simulink library "Simple_lib"  (R2018b)
settings: Solver=ode45  StartTime=0.0  StopTime=10.0  RelTol=1e-3  EnableMultiTasking=on
undefined symbols (not defined in the file or in its folder): Acceptance, beta, C, C_J, C_P, c_wall, dGain, DiscIntNeverNeededParam, Duplex, Electrical_lib, grab, h_fe, i, i3, K_T, Kman, KmanCE, mu_s, n_rev, R_arm, Simplex, systemTs, tau_0, TinIC, Ts, w_0, wallMass, Watch_lib
libraries: $bdroot x407, PlantUtilityBlockset_lib x30, peGeneralControl x22, simulink x11
(part 12 of 14)

== system Simple_lib/Hydraulic/Quadratic Heat Pipe/Push ==
  InPot : Inport
  InFlow : Inport  Tag=NOFLUX  Port=2
  FlowDisplay : Display
  Flow_PushO1BoxIIValveHydroNonStandard : Scope
      settings: Tag=Flow
  PotDisplay : Display
  Pot_PushO1BoxIIValveHydroNonStandard : Scope
      settings: Tag=Pot
  Rate Transition : RateTransition  OutPortSampleTimeMultiple=Ts  OutPortSampleTime=Ts
  OutPot : Outport  Tag=NOFLUX
  tag scope: PushO1BoxIIValveHydroNonStandard=global
  wires:
  Rate Transition/1 -> PotDisplay/1, Pot_PushO1BoxIIValveHydroNonStandard/1, OutPot/1
  InFlow/1 -> [PushO1BoxIIValveHydroNonStandard], FlowDisplay/1, Flow_PushO1BoxIIValveHydroNonStandard/1
  InPot/1 -> Rate Transition/1

== system Simple_lib/Hydraulic/Quadratic Pipe/Pull ==
  InPot : Inport  Tag=NOFLUX
  FlowDisplay : Display
  FlowGain : Gain
  FlowSum : Sum  Inputs=2  SaturateOnIntegerOverflow=on  InputSameDT=on  OutDataTypeStr=Inherit: Same as first input
  Flow_PullO1BoxIIValveHydroNonStandard : Scope
      settings: Tag=Flow
  PotDisplay : Display
  Pot_PullO1BoxIIValveHydroNonStandard : Scope
      settings: Tag=Pot
  Rate Transition : RateTransition  OutPortSampleTimeMultiple=nT  OutPortSampleTime=Ts
  OutPot : Outport
  OutFlow : Outport  Tag=NOFLUX  Port=2
  wires:
  Rate Transition/1 -> OutPot/1
  InPot/1 -> Rate Transition/1, PotDisplay/1, Pot_PullO1BoxIIValveHydroNonStandard/1
  FlowGain/1 -> OutFlow/1, Flow_PullO1BoxIIValveHydroNonStandard/1, FlowDisplay/1
  FlowSum/1 -> FlowGain/1
  [PushO3BoxXValveHydroNonStandard] -> FlowSum/1
  [PushInertiaChamber1CylinderHydroNonStandard] -> FlowSum/2

== system Simple_lib/Hydraulic/Quadratic Pipe/Push ==
  InPot : Inport
  InFlow : Inport  Tag=NOFLUX  Port=2
  FlowDisplay : Display
  Flow_PushO1BoxIIValveHydroNonStandard : Scope
      settings: Tag=Flow
  PotDisplay : Display
  Pot_PushO1BoxIIValveHydroNonStandard : Scope
      settings: Tag=Pot
  Rate Transition : RateTransition  OutPortSampleTimeMultiple=Ts  OutPortSampleTime=Ts
  OutPot : Outport  Tag=NOFLUX
  tag scope: PushO1BoxIIValveHydroNonStandard=global
  wires:
  Rate Transition/1 -> PotDisplay/1, Pot_PushO1BoxIIValveHydroNonStandard/1, OutPot/1
  InFlow/1 -> [PushO1BoxIIValveHydroNonStandard], FlowDisplay/1, Flow_PushO1BoxIIValveHydroNonStandard/1
  InPot/1 -> Rate Transition/1

== system Simple_lib/Hydraulic/Water-Glycol Heat Exchanger/Pipe1 ==
  pT_in : Inport
  Display1 : Display
  Gain : Gain  Gain=-1
  Gain1 : Gain  Gain=1e3
  I1O1BoxIIValveCannelloniHydro6 : Scope
  Product : Product  Inputs=***//  RndMeth=Zero
  Pull : Subsystem  Tag=Electrical  AncestorBlock=PlantUtilityBlockset_lib/Utility/Pull  InitFcn=initDuplex
      mask Display:
      | color('white')
      | plot([0 3], [2 2])
      | plot([0 3], [-2 -2])
      | color('black')
      | 
      | plot([0 1 1], [0 0 0.4])
      | plot([1 1 3], [0.6 1 1])
      | plot([1 3 2 1 0 2], [0.6 0.6 0.4 0.6 0.4 0.4])
      | patch([0 2 1],[0.4 0.4 0.6],[0,0,0])
      | plot([3 2 2], [1 1 0.6])
      | plot([2 2 3], [0.4 -1 -1])
  Push : Subsystem  AncestorBlock=PlantUtilityBlockset_lib/Utility/Push  InitFcn=initSimplex
      mask Display:
      | color('white')
      | plot([0 3], [2 2])
      | plot([0 3], [-2 -2])
      | color('black')
      | 
      | plot([0 2 2 3], [1 1 0 0])
      | plot([1 3 2 1 0 2], [0.6 0.6 0.4 0.6 0.4 0.4])
      | patch([1 3 2],[0.6 0.6 0.4],[0,0,0])
      | plot([0 1 1], [1 1 0.6])
      | plot([1 1 0], [0.4 -1 -1])
  Sign : Signum
  Sum : Sum  Inputs=|++
  area : Gain  Gain=0.1
  area offset : Constant  Value=0.1
  pT_out : Outport
  wires:
  Push/1(OutPot) -> Sum/1
  Sum/1 -> Pull/1(InPot)
  Gain/1 -> Sum/2
  Product/1 -> Gain1/1
  Pull/2(OutFlow) -> Display1/1, I1O1BoxIIValveCannelloniHydro6/1, Product/1, Push/2(InFlow), Sign/1, Product/3
  area offset/1 -> area/1
  Sign/1 -> Product/2
  Gain1/1 -> Gain/1
  area/1 -> Product/5, Product/4
  Pull/1(OutPot) -> pT_out/1
  pT_in/1 -> Push/1(InPot)

== system Simple_lib/Hydraulic/Water-Glycol Heat Exchanger/Pipe2 ==
  pT_in : Inport
  Display1 : Display
  Gain : Gain  Gain=-1
  Gain1 : Gain  Gain=1e3
  I1O1BoxIIValveCannelloniHydro6 : Scope
  Product : Product  Inputs=***//  RndMeth=Zero
  Pull : Subsystem  Tag=Electrical  AncestorBlock=PlantUtilityBlockset_lib/Utility/Pull  InitFcn=initDuplex
      mask Display:
      | color('white')
      | plot([0 3], [2 2])
      | plot([0 3], [-2 -2])
      | color('black')
      | 
      | plot([0 1 1], [0 0 0.4])
      | plot([1 1 3], [0.6 1 1])
      | plot([1 3 2 1 0 2], [0.6 0.6 0.4 0.6 0.4 0.4])
      | patch([0 2 1],[0.4 0.4 0.6],[0,0,0])
      | plot([3 2 2], [1 1 0.6])
      | plot([2 2 3], [0.4 -1 -1])
  Push : Subsystem  AncestorBlock=PlantUtilityBlockset_lib/Utility/Push  InitFcn=initSimplex
      mask Display:
      | color('white')
      | plot([0 3], [2 2])
      | plot([0 3], [-2 -2])
      | color('black')
      | 
      | plot([0 2 2 3], [1 1 0 0])
      | plot([1 3 2 1 0 2], [0.6 0.6 0.4 0.6 0.4 0.4])
      | patch([1 3 2],[0.6 0.6 0.4],[0,0,0])
      | plot([0 1 1], [1 1 0.6])
      | plot([1 1 0], [0.4 -1 -1])
  Sign : Signum
  Sum : Sum  Inputs=|++
  area : Gain  Gain=0.1
  area offset : Constant  Value=0.1
  pT_out : Outport
  wires:
  Push/1(OutPot) -> Sum/1
  Sum/1 -> Pull/1(InPot)
  Gain/1 -> Sum/2
  Product/1 -> Gain1/1
  Pull/2(OutFlow) -> Display1/1, I1O1BoxIIValveCannelloniHydro6/1, Product/1, Push/2(InFlow), Sign/1, Product/3
  area offset/1 -> area/1
  Sign/1 -> Product/2
  Gain1/1 -> Gain/1
  area/1 -> Product/5, Product/4
  Pull/1(OutPot) -> pT_out/1
  pT_in/1 -> Push/1(InPot)

== system Simple_lib/Hydraulic/X Heat Exchanger/Pipe1 ==
  pT_in : Inport
  Display1 : Display
  Gain : Gain  Gain=-1
  Gain1 : Gain  Gain=1e3
  I1O1BoxIIValveCannelloniHydro6 : Scope
  Product : Product  Inputs=***//  RndMeth=Zero
  Pull : Subsystem  Tag=Electrical  AncestorBlock=PlantUtilityBlockset_lib/Utility/Pull  InitFcn=initDuplex
      mask Display:
      | color('white')
      | plot([0 3], [2 2])
      | plot([0 3], [-2 -2])
      | color('black')
      | 
      | plot([0 1 1], [0 0 0.4])
      | plot([1 1 3], [0.6 1 1])
      | plot([1 3 2 1 0 2], [0.6 0.6 0.4 0.6 0.4 0.4])
      | patch([0 2 1],[0.4 0.4 0.6],[0,0,0])
      | plot([3 2 2], [1 1 0.6])
      | plot([2 2 3], [0.4 -1 -1])
  Push : Subsystem  AncestorBlock=PlantUtilityBlockset_lib/Utility/Push  InitFcn=initSimplex
      mask Display:
      | color('white')
      | plot([0 3], [2 2])
      | plot([0 3], [-2 -2])
      | color('black')
      | 
      | plot([0 2 2 3], [1 1 0 0])
      | plot([1 3 2 1 0 2], [0.6 0.6 0.4 0.6 0.4 0.4])
      | patch([1 3 2],[0.6 0.6 0.4],[0,0,0])
      | plot([0 1 1], [1 1 0.6])
      | plot([1 1 0], [0.4 -1 -1])
  Sign : Signum
  Sum : Sum  Inputs=|++
  area : Gain  Gain=0.1
  area offset : Constant  Value=0.1
  pT_out : Outport
  wires:
  pT_in/1 -> Push/1(InPot)
  Pull/1(OutPot) -> pT_out/1
  area/1 -> Product/4, Product/5
  Gain1/1 -> Gain/1
  Sign/1 -> Product/2
  area offset/1 -> area/1
  Pull/2(OutFlow) -> Product/3, Sign/1, Push/2(InFlow), Product/1, I1O1BoxIIValveCannelloniHydro6/1, Display1/1
  Product/1 -> Gain1/1
  Gain/1 -> Sum/2
  Sum/1 -> Pull/1(InPot)
  Push/1(OutPot) -> Sum/1

== system Simple_lib/Hydraulic/X Heat Exchanger/Pipe2 ==
  pT_in : Inport
  Display1 : Display
  Gain : Gain  Gain=-1
  Gain1 : Gain  Gain=1e3
  I1O1BoxIIValveCannelloniHydro6 : Scope
  Product : Product  Inputs=***//  RndMeth=Zero
  Pull : Subsystem  Tag=Electrical  AncestorBlock=PlantUtilityBlockset_lib/Utility/Pull  InitFcn=initDuplex
      mask Display:
      | color('white')
      | plot([0 3], [2 2])
      | plot([0 3], [-2 -2])
      | color('black')
      | 
      | plot([0 1 1], [0 0 0.4])
      | plot([1 1 3], [0.6 1 1])
      | plot([1 3 2 1 0 2], [0.6 0.6 0.4 0.6 0.4 0.4])
      | patch([0 2 1],[0.4 0.4 0.6],[0,0,0])
      | plot([3 2 2], [1 1 0.6])
      | plot([2 2 3], [0.4 -1 -1])
  Push : Subsystem  AncestorBlock=PlantUtilityBlockset_lib/Utility/Push  InitFcn=initSimplex
      mask Display:
      | color('white')
      | plot([0 3], [2 2])
      | plot([0 3], [-2 -2])
      | color('black')
      | 
      | plot([0 2 2 3], [1 1 0 0])
      | plot([1 3 2 1 0 2], [0.6 0.6 0.4 0.6 0.4 0.4])
      | patch([1 3 2],[0.6 0.6 0.4],[0,0,0])
      | plot([0 1 1], [1 1 0.6])
      | plot([1 1 0], [0.4 -1 -1])
  Sign : Signum
  Sum : Sum  Inputs=|++
  area : Gain  Gain=0.1
  area offset : Constant  Value=0.1
  pT_out : Outport
  wires:
  pT_in/1 -> Push/1(InPot)
  Pull/1(OutPot) -> pT_out/1
  area/1 -> Product/4, Product/5
  Gain1/1 -> Gain/1
  Sign/1 -> Product/2
  area offset/1 -> area/1
  Pull/2(OutFlow) -> Product/3, Sign/1, Push/2(InFlow), Product/1, I1O1BoxIIValveCannelloniHydro6/1, Display1/1
  Product/1 -> Gain1/1
  Gain/1 -> Sum/2
  Sum/1 -> Pull/1(InPot)
  Push/1(OutPot) -> Sum/1

== system Simple_lib/Junkyard/CinWall/C ==
  In1 : Inport
  Discrete-Time Integrator1 : DiscreteIntegrator  gainval=1/C  InitialCondition=273+TinIC  SampleTime=Ts  ICPrevOutput=DiscIntNeverNeededParam  ICPrevScaledInput=DiscIntNeverNeededParam
  Duplex : Subsystem  Tag=Electrical  AncestorBlock=PlantUtilityBlockset_lib/Utility/Duplex  InitFcn=initDuplex
      mask Display:
      | color('white')
      | plot([0 3], [2 2])
      | plot([0 3], [-2 -2])
      | color('black')
      | 
      | plot([0 1 1], [0 0 0.4])
      | plot([1 1 3], [0.6 1 1])
      | plot([1 3 2 1 0 2], [0.6 0.6 0.4 0.6 0.4 0.4])
      | patch([0 2 1],[0.4 0.4 0.6],[0,0,0])
      | plot([3 2 2], [1 1 0.6])
      | plot([2 2 3], [0.4 -1 -1])
  Simplex : Subsystem  Tag=Electrical  AncestorBlock=PlantUtilityBlockset_lib/Utility/Simplex  InitFcn=initSimplex
      mask Display:
      | color('white')
      | plot([0 3], [2 2])
      | plot([0 3], [-2 -2])
      | color('black')
      | 
      | plot([0 2 2 3], [1 1 0 0])
      | plot([1 3 2 1 0 2], [0.6 0.6 0.4 0.6 0.4 0.4])
      | patch([1 3 2],[0.6 0.6 0.4],[0,0,0])
      | plot([0 1 1], [1 1 0.6])
      | plot([1 1 0], [0.4 -1 -1])
  Sum : Sum  Inputs=|++
  Out1 : Outport
  wires:
  Sum/1 -> Duplex/1(InPot)
  Simplex/1(OutPot) -> Sum/1
  Duplex/2(OutFlow) -> Simplex/2(InFlow), Discrete-Time Integrator1/1
  Duplex/1(OutPot) -> Out1/1
  In1/1 -> Simplex/1(InPot)
  Discrete-Time Integrator1/1 -> Sum/2

== system Simple_lib/Junkyard/CinWall/Gnd ==
  Duplex : Subsystem  Tag=Electrical  AncestorBlock=PlantUtilityBlockset_lib/Utility/Duplex  InitFcn=initDuplex
      mask Display:
      | color('white')
      | plot([0 3], [2 2])
      | plot([0 3], [-2 -2])
      | color('black')
      | 
      | plot([0 1 1], [0 0 0.4])
      | plot([1 1 3], [0.6 1 1])
      | plot([1 3 2 1 0 2], [0.6 0.6 0.4 0.6 0.4 0.4])
      | patch([0 2 1],[0.4 0.4 0.6],[0,0,0])
      | plot([3 2 2], [1 1 0.6])
      | plot([2 2 3], [0.4 -1 -1])
  Ground : Ground
  Terminator : Terminator
  Out1 : Outport
  wires:
  Duplex/1(OutPot) -> Out1/1
  Ground/1 -> Duplex/1(InPot)
  Duplex/2(OutFlow) -> Terminator/1

== system Simple_lib/Junkyard/R13/Duplex ==
  InPot : Inport  Tag=NOFLUX
  FlowDisplay : Display
  FlowGain : Gain
  Flow_DuplexR13HouseWithIcons : Scope
      settings: Tag=Flow
  PotDisplay : Display
  Pot_DuplexR13HouseWithIcons : Scope
      settings: Tag=Pot
  Rate Transition : RateTransition  OutPortSampleTimeMultiple=nT  OutPortSampleTime=Ts
  OutPot : Outport
  OutFlow : Outport  Tag=NOFLUX  Port=2
  wires:
  [Simplex1R17HouseWithIcons] -> FlowGain/1
  FlowGain/1 -> FlowDisplay/1, Flow_DuplexR13HouseWithIcons/1, OutFlow/1
  InPot/1 -> Pot_DuplexR13HouseWithIcons/1, PotDisplay/1, Rate Transition/1
  Rate Transition/1 -> OutPot/1

== system Simple_lib/Junkyard/R13/Simplex ==
  InPot : Inport
  InFlow : Inport  Tag=NOFLUX  Port=2
  FlowDisplay : Display
  Flow_SimplexR13HouseWithIcons : Scope
      settings: Tag=Flow
  PotDisplay : Display
  Pot_SimplexR13HouseWithIcons : Scope
      settings: Tag=Pot
  Rate Transition : RateTransition  OutPortSampleTimeMultiple=Ts  OutPortSampleTime=Ts
  OutPot : Outport  Tag=NOFLUX
  tag scope: SimplexR13HouseWithIcons=global
  wires:
  InPot/1 -> Rate Transition/1
  InFlow/1 -> Flow_SimplexR13HouseWithIcons/1, FlowDisplay/1, [SimplexR13HouseWithIcons]
  Rate Transition/1 -> OutPot/1, Pot_SimplexR13HouseWithIcons/1, PotDisplay/1

== system Simple_lib/Junkyard/R17/Simplex ==
  InPot : Inport
  InFlow : Inport  Tag=NOFLUX  Port=2
  FlowDisplay : Display
  Flow_SimplexR17HouseWithIcons : Scope
      settings: Tag=Flow
  PotDisplay : Display
  Pot_SimplexR17HouseWithIcons : Scope
      settings: Tag=Pot
  Rate Transition : RateTransition  OutPortSampleTimeMultiple=Ts  OutPortSampleTime=Ts
  OutPot : Outport  Tag=NOFLUX
  tag scope: SimplexR17HouseWithIcons=global
  wires:
  Rate Transition/1 -> PotDisplay/1, Pot_SimplexR17HouseWithIcons/1, OutPot/1
  InFlow/1 -> [SimplexR17HouseWithIcons], FlowDisplay/1, Flow_SimplexR17HouseWithIcons/1
  InPot/1 -> Rate Transition/1

== system Simple_lib/Junkyard/R17/Simplex1 ==
  InPot : Inport
  InFlow : Inport  Tag=NOFLUX  Port=2
  FlowDisplay : Display
  Flow_Simplex1R17HouseWithIcons : Scope
      settings: Tag=Flow
  PotDisplay : Display
  Pot_Simplex1R17HouseWithIcons : Scope
      settings: Tag=Pot
  Rate Transition : RateTransition  OutPortSampleTimeMultiple=Ts  OutPortSampleTime=Ts
  OutPot : Outport  Tag=NOFLUX
  tag scope: Simplex1R17HouseWithIcons=global
  wires:
  Rate Transition/1 -> PotDisplay/1, Pot_Simplex1R17HouseWithIcons/1, OutPot/1
  InFlow/1 -> [Simplex1R17HouseWithIcons], FlowDisplay/1, Flow_Simplex1R17HouseWithIcons/1
  InPot/1 -> Rate Transition/1

== system Simple_lib/Junkyard/ThermoMeter/PushBack ==
  InPot : Inport
  InFlow : Inport  Tag=NOFLUX  Port=2
  FlowDisplay : Display
  Flow_PushBack1OilPumpFessSchematicSimulink : Scope
      settings: Tag=Flow
  PotDisplay : Display
  Pot_PushBack1OilPumpFessSchematicSimulink : Scope
      settings: Tag=Pot
  Rate Transition : RateTransition  OutPortSampleTimeMultiple=Ts  OutPortSampleTime=Ts
  OutPot : Outport  Tag=NOFLUX
  tag scope: PushBack1OilPumpFessSchematicSimulink=global
  wires:
  Rate Transition/1 -> PotDisplay/1, Pot_PushBack1OilPumpFessSchematicSimulink/1, OutPot/1
  InFlow/1 -> [PushBack1OilPumpFessSchematicSimulink], FlowDisplay/1, Flow_PushBack1OilPumpFessSchematicSimulink/1
  InPot/1 -> Rate Transition/1

== system Simple_lib/Rotational/Friction/Calculate Slip ==
  w_pos : Inport
  w_neg : Inport  Port=2
  Abs : Abs
  Abs1 : Abs
  Ground1 : Ground
  Multiply4 : Product  Inputs=*/
  Sum : Sum  Inputs=+|-
  Sum2 : Sum  Inputs=+|+
  Switch : Switch  Criteria=u2 ~= 0
  slip : Outport
  wires:
  Switch/1 -> slip/1  "slip"
  Abs1/1 -> Sum2/2
  Abs/1 -> Sum2/1
  Multiply4/1 -> Switch/1  "c"
  w_neg/1 -> Sum/2, Abs1/1
  w_pos/1 -> Abs/1, Sum/1
  Ground1/1 -> Switch/3
  Sum/1 -> Multiply4/1  "dtheta"
  Sum2/1 -> Switch/2, Multiply4/2  "denom"

== system Simple_lib/Rotational/Friction/Derivative ==
  y : Inport
  x : Inport  Port=2
  Abs : Abs
  Divide : Product  Inputs=*/
  Ground{1..4} (4 alike) : Ground
  Integrator (Discrete or Continuous)1 : peGeneralControl/Integrator (Discrete or Continuous)  LabelModeActiveChoice=Discrete  ExternalReset=level  LimitType=Anti-windup  B=inf  A=-inf  Ts=-1
  Integrator (Discrete or Continuous)2 : peGeneralControl/Integrator (Discrete or Continuous)  LabelModeActiveChoice=Discrete  ExternalReset=level  LimitType=Anti-windup  B=inf  A=-inf  Ts=-1
  Saturation : Saturate  UpperLimit=inf  LowerLimit=-inf
  Sum1 : Sum  Inputs=|+-
  Sum2 : Sum  Inputs=|+-
  Switch : Switch  Criteria=u2 > Threshold  Threshold=1e-6
  Unit Delay : UnitDelay  SampleTime=-1
  Weighted Sample Time1 : SampleTimeMath  TsampMathOp=/  weightValue=1
  Weighted Sample Time3 : SampleTimeMath  TsampMathOp=/  weightValue=1
  dy/dx : Outport
  wires:
  Divide/1 -> Switch/1
  Switch/1 -> Saturation/1
  Unit Delay/1 -> Switch/3
  Saturation/1 -> Unit Delay/1, dy/dx/1
  Abs/1 -> Switch/2
  Weighted Sample Time3/1 -> Divide/1, Integrator (Discrete or Continuous)1/1  "dI"
  Ground3/1 -> Integrator (Discrete or Continuous)1/3
  Sum1/1 -> Weighted Sample Time3/1
  Ground2/1 -> Integrator (Discrete or Continuous)1/2
  Integrator (Discrete or Continuous)1/1 -> Sum1/2
  y/1 -> Sum1/1
  Weighted Sample Time1/1 -> Divide/2, Abs/1, Integrator (Discrete or Continuous)2/1  "dI"
  Ground4/1 -> Integrator (Discrete or Continuous)2/3
  Sum2/1 -> Weighted Sample Time1/1
  Ground1/1 -> Integrator (Discrete or Continuous)2/2
  Integrator (Discrete or Continuous)2/1 -> Sum2/2
  x/1 -> Sum2/1

== system Simple_lib/Rotational/Friction/Gaussian Spring ==
  slip : Inport
  Exp : Math  SaturateOnIntegerOverflow=on
  Gain : Gain  Gain=-1/2
  Ground2 : Ground
  Ground3 : Ground
  Integrator (Discrete or Continuous)1 : peGeneralControl/Integrator (Discrete or Continuous)  LabelModeActiveChoice=Discrete  ExternalReset=level  LimitType=Anti-windup  B=inf  A=-inf  Ts=-1
  Multiply1 : Product  Inputs=/*
  Multiply2 : Product  Inputs=/**
  Square : Math  Operator=square  SaturateOnIntegerOverflow=on
  Square1 : Math  Operator=square  SaturateOnIntegerOverflow=on
  normalise : Gain  Gain=1/sqrt(2*pi)
  sigma : Constant  Value=s
  tau : Outport
  wires:
  Ground2/1 -> Integrator (Discrete or Continuous)1/2
  Ground3/1 -> Integrator (Discrete or Continuous)1/3
  normalise/1 -> tau/1
  Square/1 -> Multiply1/2
  sigma/1 -> Multiply2/1, Square1/1
  Integrator (Discrete or Continuous)1/1 -> normalise/1  "theta"
  slip/1 -> Multiply2/3, Square/1
  Multiply2/1 -> Integrator (Discrete or Continuous)1/1  "gauss"
  Multiply1/1 -> Gain/1  "stds"
  Exp/1 -> Multiply2/2
  Square1/1 -> Multiply1/1
  Gain/1 -> Exp/1

== system Simple_lib/Thermal/CinWall/C ==
  In1 : Inport
  Discrete-Time Integrator1 : DiscreteIntegrator  gainval=1/C  InitialCondition=273+TinIC  SampleTime=Ts  ICPrevOutput=DiscIntNeverNeededParam  ICPrevScaledInput=DiscIntNeverNeededParam
  Duplex : Subsystem  Tag=Electrical  AncestorBlock=PlantUtilityBlockset_lib/Utility/Duplex  InitFcn=initDuplex
      mask Display:
      | color('white')
      | plot([0 3], [2 2])
      | plot([0 3], [-2 -2])
      | color('black')
      | 
      | plot([0 1 1], [0 0 0.4])
      | plot([1 1 3], [0.6 1 1])
      | plot([1 3 2 1 0 2], [0.6 0.6 0.4 0.6 0.4 0.4])
      | patch([0 2 1],[0.4 0.4 0.6],[0,0,0])
      | plot([3 2 2], [1 1 0.6])
      | plot([2 2 3], [0.4 -1 -1])
  Simplex : Subsystem  Tag=Electrical  AncestorBlock=PlantUtilityBlockset_lib/Utility/Simplex  InitFcn=initSimplex
      mask Display:
      | color('white')
      | plot([0 3], [2 2])
      | plot([0 3], [-2 -2])
      | color('black')
      | 
      | plot([0 2 2 3], [1 1 0 0])
      | plot([1 3 2 1 0 2], [0.6 0.6 0.4 0.6 0.4 0.4])
      | patch([1 3 2],[0.6 0.6 0.4],[0,0,0])
      | plot([0 1 1], [1 1 0.6])
      | plot([1 1 0], [0.4 -1 -1])
  Sum : Sum  Inputs=|++
  Out1 : Outport
  wires:
  Sum/1 -> Duplex/1(InPot)
  Simplex/1(OutPot) -> Sum/1
  Duplex/2(OutFlow) -> Simplex/2(InFlow), Discrete-Time Integrator1/1
  Duplex/1(OutPot) -> Out1/1
  In1/1 -> Simplex/1(InPot)
  Discrete-Time Integrator1/1 -> Sum/2

== system Simple_lib/Thermal/CinWall/Gnd ==
  Duplex : Subsystem  Tag=Electrical  AncestorBlock=PlantUtilityBlockset_lib/Utility/Duplex  InitFcn=initDuplex
      mask Display:
      | color('white')
      | plot([0 3], [2 2])
      | plot([0 3], [-2 -2])
      | color('black')
      | 
      | plot([0 1 1], [0 0 0.4])
      | plot([1 1 3], [0.6 1 1])
      | plot([1 3 2 1 0 2], [0.6 0.6 0.4 0.6 0.4 0.4])
      | patch([0 2 1],[0.4 0.4 0.6],[0,0,0])
      | plot([3 2 2], [1 1 0.6])
      | plot([2 2 3], [0.4 -1 -1])
  Ground : Ground
  Terminator : Terminator
  Out1 : Outport
  wires:
  Duplex/1(OutPot) -> Out1/1
  Ground/1 -> Duplex/1(InPot)
  Duplex/2(OutFlow) -> Terminator/1

== system Simple_lib/Thermal/R13/Duplex ==
  InPot : Inport  Tag=NOFLUX
  FlowDisplay : Display
  FlowGain : Gain
  Flow_DuplexR13HouseWithIcons : Scope
      settings: Tag=Flow
  PotDisplay : Display
  Pot_DuplexR13HouseWithIcons : Scope
      settings: Tag=Pot
  Rate Transition : RateTransition  OutPortSampleTimeMultiple=nT  OutPortSampleTime=Ts
  OutPot : Outport
  OutFlow : Outport  Tag=NOFLUX  Port=2
  wires:
  [Simplex1R17HouseWithIcons] -> FlowGain/1
  FlowGain/1 -> FlowDisplay/1, Flow_DuplexR13HouseWithIcons/1, OutFlow/1
  InPot/1 -> Pot_DuplexR13HouseWithIcons/1, PotDisplay/1, Rate Transition/1
  Rate Transition/1 -> OutPot/1

== system Simple_lib/Thermal/R13/Simplex ==
  InPot : Inport
  InFlow : Inport  Tag=NOFLUX  Port=2
  FlowDisplay : Display
  Flow_SimplexR13HouseWithIcons : Scope
      settings: Tag=Flow
  PotDisplay : Display
  Pot_SimplexR13HouseWithIcons : Scope
      settings: Tag=Pot
  Rate Transition : RateTransition  OutPortSampleTimeMultiple=Ts  OutPortSampleTime=Ts
  OutPot : Outport  Tag=NOFLUX
  tag scope: SimplexR13HouseWithIcons=global
  wires:
  InPot/1 -> Rate Transition/1
  InFlow/1 -> Flow_SimplexR13HouseWithIcons/1, FlowDisplay/1, [SimplexR13HouseWithIcons]
  Rate Transition/1 -> OutPot/1, Pot_SimplexR13HouseWithIcons/1, PotDisplay/1

== system Simple_lib/Thermal/R17/Simplex ==
  InPot : Inport
  InFlow : Inport  Tag=NOFLUX  Port=2
  FlowDisplay : Display
  Flow_SimplexR17HouseWithIcons : Scope
      settings: Tag=Flow
  PotDisplay : Display
  Pot_SimplexR17HouseWithIcons : Scope
      settings: Tag=Pot
  Rate Transition : RateTransition  OutPortSampleTimeMultiple=Ts  OutPortSampleTime=Ts
  OutPot : Outport  Tag=NOFLUX
  tag scope: SimplexR17HouseWithIcons=global
  wires:
  Rate Transition/1 -> PotDisplay/1, Pot_SimplexR17HouseWithIcons/1, OutPot/1
  InFlow/1 -> [SimplexR17HouseWithIcons], FlowDisplay/1, Flow_SimplexR17HouseWithIcons/1
  InPot/1 -> Rate Transition/1

== system Simple_lib/Thermal/R17/Simplex1 ==
  InPot : Inport
  InFlow : Inport  Tag=NOFLUX  Port=2
  FlowDisplay : Display
  Flow_Simplex1R17HouseWithIcons : Scope
      settings: Tag=Flow
  PotDisplay : Display
  Pot_Simplex1R17HouseWithIcons : Scope
      settings: Tag=Pot
  Rate Transition : RateTransition  OutPortSampleTimeMultiple=Ts  OutPortSampleTime=Ts
  OutPot : Outport  Tag=NOFLUX
  tag scope: Simplex1R17HouseWithIcons=global
  wires:
  Rate Transition/1 -> PotDisplay/1, Pot_Simplex1R17HouseWithIcons/1, OutPot/1
  InFlow/1 -> [Simplex1R17HouseWithIcons], FlowDisplay/1, Flow_Simplex1R17HouseWithIcons/1
  InPot/1 -> Rate Transition/1

== system Simple_lib/Thermal/ThermoMeter/PushBack ==
  InPot : Inport
  InFlow : Inport  Tag=NOFLUX  Port=2
  FlowDisplay : Display
  Flow_PushBack1OilPumpFessSchematicSimulink : Scope
      settings: Tag=Flow
  PotDisplay : Display
  Pot_PushBack1OilPumpFessSchematicSimulink : Scope
      settings: Tag=Pot
  Rate Transition : RateTransition  OutPortSampleTimeMultiple=Ts  OutPortSampleTime=Ts
  OutPot : Outport  Tag=NOFLUX
  tag scope: PushBack1OilPumpFessSchematicSimulink=global
  wires:
  Rate Transition/1 -> PotDisplay/1, Pot_PushBack1OilPumpFessSchematicSimulink/1, OutPot/1
  InFlow/1 -> [PushBack1OilPumpFessSchematicSimulink], FlowDisplay/1, Flow_PushBack1OilPumpFessSchematicSimulink/1
  InPot/1 -> Rate Transition/1

== system Simple_lib/Driveline/Changan Transmission/EMachine/J_eMotor ==
  Discrete-Time Integrator1 : DiscreteIntegrator  gainval=1/1  SampleTime=Ts  ICPrevOutput=DiscIntNeverNeededParam  ICPrevScaledInput=DiscIntNeverNeededParam
  Pull : Subsystem  Tag=Electrical  AncestorBlock=PlantUtilityBlockset_lib/Utility/Pull  InitFcn=initDuplex
      mask Display:
      | color('white')
      | plot([0 3], [2 2])
      | plot([0 3], [-2 -2])
      | color('black')
      | 
      | plot([0 1 1], [0 0 0.4])
      | plot([1 1 3], [0.6 1 1])
      | plot([1 3 2 1 0 2], [0.6 0.6 0.4 0.6 0.4 0.4])
      | patch([0 2 1],[0.4 0.4 0.6],[0,0,0])
      | plot([3 2 2], [1 1 0.6])
      | plot([2 2 3], [0.4 -1 -1])
  Out1 : Outport
  wires:
  Discrete-Time Integrator1/1 -> Pull/1(InPot)
  Pull/2(OutFlow) -> Discrete-Time Integrator1/1
  Pull/1(OutPot) -> Out1/1

== system Simple_lib/Driveline/Changan Transmission/EMachine/Transducer ==
  w : Inport
  Duplex : Subsystem  Tag=Electrical  AncestorBlock=PlantUtilityBlockset_lib/Utility/Pull  InitFcn=initDuplex
      mask Display:
      | color('white')
      | plot([0 3], [2 2])
      | plot([0 3], [-2 -2])
      | color('black')
      | 
      | plot([0 1 1], [0 0 0.4])
      | plot([1 1 3], [0.6 1 1])
      | plot([1 3 2 1 0 2], [0.6 0.6 0.4 0.6 0.4 0.4])
      | patch([0 2 1],[0.4 0.4 0.6],[0,0,0])
      | plot([3 2 2], [1 1 0.6])
      | plot([2 2 3], [0.4 -1 -1])
  Simplex : Subsystem  Tag=Electrical  AncestorBlock=PlantUtilityBlockset_lib/Utility/Push  InitFcn=initSimplex
      mask Display:
      | color('white')
      | plot([0 3], [2 2])
      | plot([0 3], [-2 -2])
      | color('black')
      | 
      | plot([0 2 2 3], [1 1 0 0])
      | plot([1 3 2 1 0 2], [0.6 0.6 0.4 0.6 0.4 0.4])
      | patch([1 3 2],[0.6 0.6 0.4],[0,0,0])
      | plot([0 1 1], [1 1 0.6])
      | plot([1 1 0], [0.4 -1 -1])
  Torque Constant = 60/2/pi/K_V : Gain  Gain=K_T
  Torque Constant K_T : Gain  Gain=K_T
  V : Outport
  wires:
  Torque Constant = 60/2/pi/K_V/1 -> Duplex/1(InPot)
  Duplex/2(OutFlow) -> Torque Constant K_T/1  "I"
  w/1 -> Simplex/1(InPot)
  Duplex/1(OutPot) -> V/1
  Simplex/1(OutPot) -> Torque Constant = 60/2/pi/K_V/1
  Torque Constant K_T/1 -> Simplex/2(InFlow)  "tau"

== system Simple_lib/Driveline/Changan Transmission/FD1/Pull ==
  InPot : Inport  Tag=NOFLUX
  FlowGain : Gain
  FlowSum : Sum  Inputs=3  SaturateOnIntegerOverflow=on  InputSameDT=on  OutDataTypeStr=Inherit: Same as first input
  OutPot : Outport
  OutFlow : Outport  Tag=NOFLUX  Port=2
  wires:
  InPot/1 -> OutPot/1  "p_DuplexInverter_test0"
  FlowGain/1 -> OutFlow/1  "f_DuplexInverter_test0"
  FlowSum/1 -> FlowGain/1
  [Push_inSynchro3TransmissionHYBPTPlantHybpt_test] -> FlowSum/1
  [Push_inSynchro5TransmissionHYBPTPlantHybpt_test] -> FlowSum/2
  [Push_inSynchro6TransmissionHYBPTPlantHybpt_test] -> FlowSum/3

== system Simple_lib/Driveline/Changan Transmission/FD1/Push ==
  InPot : Inport
  InFlow : Inport  Tag=NOFLUX  Port=2
  OutPot : Outport  Tag=NOFLUX
  tag scope: PushFD1TransmissionHYBPTPlantHybpt_test=global
  wires:
  InFlow/1 -> [PushFD1TransmissionHYBPTPlantHybpt_test]  "flow"
  InPot/1 -> OutPot/1  "pot"

== system Simple_lib/Driveline/Changan Transmission/FD2/Pull ==
  InPot : Inport  Tag=NOFLUX
  FlowGain : Gain
  FlowSum : Sum  Inputs=4  SaturateOnIntegerOverflow=on  InputSameDT=on  OutDataTypeStr=Inherit: Same as first input
  OutPot : Outport
  OutFlow : Outport  Tag=NOFLUX  Port=2
  wires:
  InPot/1 -> OutPot/1  "p_DuplexInverter_test0"
  FlowGain/1 -> OutFlow/1  "f_DuplexInverter_test0"
  FlowSum/1 -> FlowGain/1
  [Push_inSynchroTransmissionHYBPTPlantHybpt_test] -> FlowSum/1
  [Push_inSynchro4TransmissionHYBPTPlantHybpt_test] -> FlowSum/2
  [Push_inSynchro2TransmissionHYBPTPlantHybpt_test] -> FlowSum/3
  [Push_inSynchro1TransmissionHYBPTPlantHybpt_test] -> FlowSum/4

== system Simple_lib/Driveline/Changan Transmission/FD2/Push ==
  InPot : Inport
  InFlow : Inport  Tag=NOFLUX  Port=2
  OutPot : Outport  Tag=NOFLUX
  tag scope: PushFD2TransmissionHYBPTPlantHybpt_test=global
  wires:
  InFlow/1 -> [PushFD2TransmissionHYBPTPlantHybpt_test]  "flow"
  InPot/1 -> OutPot/1  "pot"

== system Simple_lib/Driveline/Changan Transmission/GP1/Pull ==
  InPot : Inport  Tag=NOFLUX
  FlowGain : Gain
  OutPot : Outport
  OutFlow : Outport  Tag=NOFLUX  Port=2
  wires:
  InPot/1 -> OutPot/1  "p_DuplexInverter_test0"
  FlowGain/1 -> OutFlow/1  "f_DuplexInverter_test0"
  [Push_outSynchro3TransmissionHYBPTPlantHybpt_test] -> FlowGain/1

== system Simple_lib/Driveline/Changan Transmission/GP1/Push ==
  InPot : Inport
  InFlow : Inport  Tag=NOFLUX  Port=2
  OutPot : Outport  Tag=NOFLUX
  tag scope: PushGP1TransmissionHYBPTPlantHybpt_test=global
  wires:
  InFlow/1 -> [PushGP1TransmissionHYBPTPlantHybpt_test]  "flow"
  InPot/1 -> OutPot/1  "pot"

== system Simple_lib/Driveline/Changan Transmission/GP2/Pull ==
  InPot : Inport  Tag=NOFLUX
  FlowGain : Gain
  FlowSum : Sum  Inputs=2  SaturateOnIntegerOverflow=on  InputSameDT=on  OutDataTypeStr=Inherit: Same as first input
  OutPot : Outport
  OutFlow : Outport  Tag=NOFLUX  Port=2
  wires:
  InPot/1 -> OutPot/1  "p_DuplexInverter_test0"
  FlowGain/1 -> OutFlow/1  "f_DuplexInverter_test0"
  FlowSum/1 -> FlowGain/1
  [Push_outSynchroTransmissionHYBPTPlantHybpt_test] -> FlowSum/1
  [PushGPRTransmissionHYBPTPlantHybpt_test] -> FlowSum/2

== system Simple_lib/Driveline/Changan Transmission/GP2/Push ==
  InPot : Inport
  InFlow : Inport  Tag=NOFLUX  Port=2
  OutPot : Outport  Tag=NOFLUX
  tag scope: PushGP2TransmissionHYBPTPlantHybpt_test=global
  wires:
  InFlow/1 -> [PushGP2TransmissionHYBPTPlantHybpt_test]  "flow"
  InPot/1 -> OutPot/1  "pot"

== system Simple_lib/Driveline/Changan Transmission/GP3/Pull ==
  InPot : Inport  Tag=NOFLUX
  FlowGain : Gain
  OutPot : Outport
  OutFlow : Outport  Tag=NOFLUX  Port=2
  wires:
  InPot/1 -> OutPot/1  "p_DuplexInverter_test0"
  FlowGain/1 -> OutFlow/1  "f_DuplexInverter_test0"
  [Push_outSynchro2TransmissionHYBPTPlantHybpt_test] -> FlowGain/1

== system Simple_lib/Driveline/Changan Transmission/GP3/Push ==
  InPot : Inport
  InFlow : Inport  Tag=NOFLUX  Port=2
  OutPot : Outport  Tag=NOFLUX
  tag scope: PushGP3TransmissionHYBPTPlantHybpt_test=global
  wires:
  InFlow/1 -> [PushGP3TransmissionHYBPTPlantHybpt_test]  "flow"
  InPot/1 -> OutPot/1  "pot"

== system Simple_lib/Driveline/Changan Transmission/GP4 /Pull ==
  InPot : Inport  Tag=NOFLUX
  FlowGain : Gain
  OutPot : Outport
  OutFlow : Outport  Tag=NOFLUX  Port=2
  wires:
  InPot/1 -> OutPot/1  "p_DuplexInverter_test0"
  FlowGain/1 -> OutFlow/1  "f_DuplexInverter_test0"
  [Push_outSynchro5TransmissionHYBPTPlantHybpt_test] -> FlowGain/1

== system Simple_lib/Driveline/Changan Transmission/GP4 /Push ==
  InPot : Inport
  InFlow : Inport  Tag=NOFLUX  Port=2
  OutPot : Outport  Tag=NOFLUX
  tag scope: PushGP4TransmissionHYBPTPlantHybpt_test=global
  wires:
  InFlow/1 -> [PushGP4TransmissionHYBPTPlantHybpt_test]  "flow"
  InPot/1 -> OutPot/1  "pot"

== system Simple_lib/Driveline/Changan Transmission/GP5/Pull ==
  InPot : Inport  Tag=NOFLUX
  FlowGain : Gain
  OutPot : Outport
  OutFlow : Outport  Tag=NOFLUX  Port=2
  wires:
  InPot/1 -> OutPot/1  "p_DuplexInverter_test0"
  FlowGain/1 -> OutFlow/1  "f_DuplexInverter_test0"
  [Push_outSynchro1TransmissionHYBPTPlantHybpt_test] -> FlowGain/1

== system Simple_lib/Driveline/Changan Transmission/GP5/Push ==
  InPot : Inport
  InFlow : Inport  Tag=NOFLUX  Port=2
  OutPot : Outport  Tag=NOFLUX
  tag scope: PushGP5TransmissionHYBPTPlantHybpt_test=global
  wires:
  InFlow/1 -> [PushGP5TransmissionHYBPTPlantHybpt_test]  "flow"
  InPot/1 -> OutPot/1  "pot"

== system Simple_lib/Driveline/Changan Transmission/GP6/Pull ==
  InPot : Inport  Tag=NOFLUX
  FlowGain : Gain
  OutPot : Outport
  OutFlow : Outport  Tag=NOFLUX  Port=2
  wires:
  InPot/1 -> OutPot/1  "p_DuplexInverter_test0"
  FlowGain/1 -> OutFlow/1  "f_DuplexInverter_test0"
  [Push_outSynchro4TransmissionHYBPTPlantHybpt_test] -> FlowGain/1

== system Simple_lib/Driveline/Changan Transmission/GP6/Push ==
  InPot : Inport
  InFlow : Inport  Tag=NOFLUX  Port=2
  OutPot : Outport  Tag=NOFLUX
  tag scope: PushGP6TransmissionHYBPTPlantHybpt_test=global
  wires:
  InFlow/1 -> [PushGP6TransmissionHYBPTPlantHybpt_test]  "flow"
  InPot/1 -> OutPot/1  "pot"

== system Simple_lib/Driveline/Changan Transmission/GPR/Pull ==
  InPot : Inport  Tag=NOFLUX
  FlowGain : Gain
  OutPot : Outport
  OutFlow : Outport  Tag=NOFLUX  Port=2
  wires:
  InPot/1 -> OutPot/1  "p_DuplexInverter_test0"
  FlowGain/1 -> OutFlow/1  "f_DuplexInverter_test0"
  [Push_outSynchro6TransmissionHYBPTPlantHybpt_test] -> FlowGain/1

== system Simple_lib/Driveline/Changan Transmission/GPR/Push ==
  InPot : Inport
  InFlow : Inport  Tag=NOFLUX  Port=2
  OutPot : Outport  Tag=NOFLUX
  tag scope: PushGPRTransmissionHYBPTPlantHybpt_test=global
  wires:
  InFlow/1 -> [PushGPRTransmissionHYBPTPlantHybpt_test]  "flow"
  InPot/1 -> OutPot/1  "pot"

== system Simple_lib/Driveline/Changan Transmission/K0/Dynamic Friction ==
  Dw : Inport
  cap : Inport  Port=2
  Product : Product  RndMeth=Zero
  Saturation : Saturate  UpperLimit=inf  LowerLimit=0
  friction : Trigonometry  Operator=tanh
  grab : Gain  Gain=grab
  Tq_dyn : Outport
  wires:
  Dw/1 -> grab/1
  grab/1 -> friction/1
  friction/1 -> Product/1
  cap/1 -> Saturation/1
  Saturation/1 -> Product/2
  Product/1 -> Tq_dyn/1

== system Simple_lib/Driveline/Changan Transmission/K0/Push_in ==
  InPot : Inport
  InFlow : Inport  Tag=NOFLUX  Port=2
  OutPot : Outport  Tag=NOFLUX
  tag scope: Push_inK0TransmissionHYBPTPlantHybpt_test=global
  wires:
  InPot/1 -> OutPot/1  "pot"
  InFlow/1 -> [Push_inK0TransmissionHYBPTPlantHybpt_test]  "flow"

== system Simple_lib/Driveline/Changan Transmission/K0/Push_out ==
  InPot : Inport
  InFlow : Inport  Tag=NOFLUX  Port=2
  OutPot : Outport  Tag=NOFLUX
  tag scope: Push_outK0TransmissionHYBPTPlantHybpt_test=global
  wires:
  InPot/1 -> OutPot/1  "pot"
  InFlow/1 -> [Push_outK0TransmissionHYBPTPlantHybpt_test]  "flow"

== system Simple_lib/Driveline/Changan Transmission/K0/Static Friction ==
  cap : Inport
  Dw : Inport  Port=2
  w : Inport  Port=3
  Tq : Inport  Port=4
  1/R2 : Gain  Gain=mu_s/2
  Abs : Abs
  Abs1 : Abs
  Abs2 : Abs
  Delay : Delay  DelayLength=1  InitialCondition=0
  Discrete-Time Integrator : DiscreteIntegrator  gainval=k_static  ExternalReset=level  SampleTime=Ts  ICPrevOutput=DiscIntNeverNeededParam  ICPrevScaledInput=DiscIntNeverNeededParam
  Logical Operator : Logic  Operator=OR  AllPortsSameDT=off  OutDataTypeStr=boolean
  Logical Operator1 : Logic  AllPortsSameDT=off  OutDataTypeStr=boolean
  Logical Operator2 : Logic  Operator=NOT  Inputs=1  AllPortsSameDT=off  OutDataTypeStr=boolean
  Relational Operator : RelationalOperator  OutDataTypeStr=boolean  RndMeth=Nearest
  Relational Operator1 : RelationalOperator  OutDataTypeStr=boolean  RndMeth=Nearest
  Saturation1 : Saturate  UpperLimit=inf  LowerLimit=0
  Sum2 : Sum  Inputs=-++
  big speed diff : Scope
  capacity : Scope
  oldtrans_exceeds_cap : Scope
  slipping : Scope
  Tq_stat : Outport
  wires:
  1/R2/1 -> Relational Operator/2
  Relational Operator/1 -> Logical Operator/1, big speed diff/1
  cap/1 -> capacity/1, Saturation1/1
  Logical Operator/1 -> slipping/1, Discrete-Time Integrator/2
  Discrete-Time Integrator/1 -> Tq_stat/1
  Abs/1 -> Relational Operator/1
  Abs2/1 -> Relational Operator1/1
  Saturation1/1 -> Relational Operator1/2
  Abs1/1 -> 1/R2/1
  Logical Operator1/1 -> oldtrans_exceeds_cap/1, Logical Operator/2
  Sum2/1 -> Abs1/1
  Tq/1 -> Abs2/1
  w/1 -> Sum2/2, Sum2/3
  Dw/1 -> Discrete-Time Integrator/1, Abs/1, Sum2/1
  Relational Operator1/1 -> Delay/1, Logical Operator1/1
  Delay/1 -> Logical Operator2/1
  Logical Operator2/1 -> Logical Operator1/2

== system Simple_lib/Driveline/Changan Transmission/K1/Dynamic Friction ==
  Dw : Inport
  cap : Inport  Port=2
  Product : Product  RndMeth=Zero
  Saturation : Saturate  UpperLimit=inf  LowerLimit=0
  friction : Trigonometry  Operator=tanh
  grab : Gain  Gain=grab
  Tq_dyn : Outport
  wires:
  Dw/1 -> grab/1
  grab/1 -> friction/1
  friction/1 -> Product/2
  cap/1 -> Saturation/1
  Saturation/1 -> Product/1
  Product/1 -> Tq_dyn/1

== system Simple_lib/Driveline/Changan Transmission/K1/Push_in ==
  InPot : Inport
  InFlow : Inport  Tag=NOFLUX  Port=2
  OutPot : Outport  Tag=NOFLUX
  tag scope: Push_inK1TransmissionHYBPTPlantHybpt_test=global
  wires:
  InPot/1 -> OutPot/1  "pot"
  InFlow/1 -> [Push_inK1TransmissionHYBPTPlantHybpt_test]  "flow"

== system Simple_lib/Driveline/Changan Transmission/K1/Push_out ==
  InPot : Inport
  InFlow : Inport  Tag=NOFLUX  Port=2
  OutPot : Outport  Tag=NOFLUX
  tag scope: Push_outK1TransmissionHYBPTPlantHybpt_test=global
  wires:
  InPot/1 -> OutPot/1  "pot"
  InFlow/1 -> [Push_outK1TransmissionHYBPTPlantHybpt_test]  "flow"

== system Simple_lib/Driveline/Changan Transmission/K1/Static Friction ==
  cap : Inport
  Dw : Inport  Port=2
  w : Inport  Port=3
  Tq : Inport  Port=4
  1/R2 : Gain  Gain=mu_s/2
  Abs : Abs
  Abs1 : Abs
  Abs2 : Abs
  Delay : Delay  DelayLength=1  InitialCondition=0
  Discrete-Time Integrator : DiscreteIntegrator  gainval=k_static  ExternalReset=level  SampleTime=Ts  ICPrevOutput=DiscIntNeverNeededParam  ICPrevScaledInput=DiscIntNeverNeededParam
  Logical Operator : Logic  Operator=OR  AllPortsSameDT=off  OutDataTypeStr=boolean
  Logical Operator1 : Logic  AllPortsSameDT=off  OutDataTypeStr=boolean
  Logical Operator2 : Logic  Operator=NOT  Inputs=1  AllPortsSameDT=off  OutDataTypeStr=boolean
  Relational Operator : RelationalOperator  OutDataTypeStr=boolean  RndMeth=Nearest
  Relational Operator1 : RelationalOperator  OutDataTypeStr=boolean  RndMeth=Nearest
  Saturation1 : Saturate  UpperLimit=inf  LowerLimit=0
  Sum2 : Sum  Inputs=-++
  big speed diff : Scope
  capacity : Scope
  oldtrans_exceeds_cap : Scope
  slipping : Scope
  Tq_stat : Outport
  wires:
  1/R2/1 -> Relational Operator/2
  Relational Operator/1 -> Logical Operator/1, big speed diff/1
  cap/1 -> capacity/1, Saturation1/1
  Logical Operator/1 -> slipping/1, Discrete-Time Integrator/2
  Discrete-Time Integrator/1 -> Tq_stat/1
  Abs/1 -> Relational Operator/1
  Abs2/1 -> Relational Operator1/1
  Saturation1/1 -> Relational Operator1/2
  Abs1/1 -> 1/R2/1
  Logical Operator1/1 -> oldtrans_exceeds_cap/1, Logical Operator/2
  Sum2/1 -> Abs1/1
  Tq/1 -> Abs2/1
  w/1 -> Sum2/2, Sum2/3
  Dw/1 -> Discrete-Time Integrator/1, Abs/1, Sum2/1
  Relational Operator1/1 -> Delay/1, Logical Operator1/1
  Delay/1 -> Logical Operator2/1
  Logical Operator2/1 -> Logical Operator1/2

== system Simple_lib/Driveline/Changan Transmission/K2/Dynamic Friction ==
  Dw : Inport
  cap : Inport  Port=2
  Product : Product  RndMeth=Zero
  Saturation : Saturate  UpperLimit=inf  LowerLimit=0
  friction : Trigonometry  Operator=tanh
  grab : Gain  Gain=grab
  Tq_dyn : Outport
  wires:
  Dw/1 -> grab/1
  grab/1 -> friction/1
  friction/1 -> Product/2
  cap/1 -> Saturation/1
  Saturation/1 -> Product/1
  Product/1 -> Tq_dyn/1

== system Simple_lib/Driveline/Changan Transmission/K2/Push_in ==
  InPot : Inport
  InFlow : Inport  Tag=NOFLUX  Port=2
  OutPot : Outport  Tag=NOFLUX
  tag scope: Push_inK2TransmissionHYBPTPlantHybpt_test=global
  wires:
  InPot/1 -> OutPot/1  "pot"
  InFlow/1 -> [Push_inK2TransmissionHYBPTPlantHybpt_test]  "flow"

== system Simple_lib/Driveline/Changan Transmission/K2/Push_out ==
  InPot : Inport
  InFlow : Inport  Tag=NOFLUX  Port=2
  OutPot : Outport  Tag=NOFLUX
  tag scope: Push_outK2TransmissionHYBPTPlantHybpt_test=global
  wires:
  InPot/1 -> OutPot/1  "pot"
  InFlow/1 -> [Push_outK2TransmissionHYBPTPlantHybpt_test]  "flow"

== system Simple_lib/Driveline/Changan Transmission/K2/Static Friction ==
  cap : Inport
  Dw : Inport  Port=2
  w : Inport  Port=3
  Tq : Inport  Port=4
  1/R2 : Gain  Gain=mu_s/2
  Abs : Abs
  Abs1 : Abs
  Abs2 : Abs
  Delay : Delay  DelayLength=1  InitialCondition=0
  Discrete-Time Integrator : DiscreteIntegrator  gainval=k_static  ExternalReset=level  SampleTime=Ts  ICPrevOutput=DiscIntNeverNeededParam  ICPrevScaledInput=DiscIntNeverNeededParam
  Logical Operator : Logic  Operator=OR  AllPortsSameDT=off  OutDataTypeStr=boolean
  Logical Operator1 : Logic  AllPortsSameDT=off  OutDataTypeStr=boolean
  Logical Operator2 : Logic  Operator=NOT  Inputs=1  AllPortsSameDT=off  OutDataTypeStr=boolean
  Relational Operator : RelationalOperator  OutDataTypeStr=boolean  RndMeth=Nearest
  Relational Operator1 : RelationalOperator  OutDataTypeStr=boolean  RndMeth=Nearest
  Saturation1 : Saturate  UpperLimit=inf  LowerLimit=0
  Sum2 : Sum  Inputs=-++
  big speed diff : Scope
  capacity : Scope
  oldtrans_exceeds_cap : Scope
  slipping : Scope
  Tq_stat : Outport
  wires:
  1/R2/1 -> Relational Operator/2
  Relational Operator/1 -> Logical Operator/1, big speed diff/1
  cap/1 -> capacity/1, Saturation1/1
  Logical Operator/1 -> slipping/1, Discrete-Time Integrator/2
  Discrete-Time Integrator/1 -> Tq_stat/1
  Abs/1 -> Relational Operator/1
  Abs2/1 -> Relational Operator1/1
  Saturation1/1 -> Relational Operator1/2
  Abs1/1 -> 1/R2/1
  Logical Operator1/1 -> oldtrans_exceeds_cap/1, Logical Operator/2
  Sum2/1 -> Abs1/1
  Tq/1 -> Abs2/1
  w/1 -> Sum2/2, Sum2/3
  Dw/1 -> Discrete-Time Integrator/1, Abs/1, Sum2/1
  Relational Operator1/1 -> Delay/1, Logical Operator1/1
  Delay/1 -> Logical Operator2/1
  Logical Operator2/1 -> Logical Operator1/2

== system Simple_lib/Driveline/Changan Transmission/LoadScopes/Pull ==
  InPot : Inport  Tag=NOFLUX
  FlowGain : Gain
  FlowSum : Sum  Inputs=2  SaturateOnIntegerOverflow=on  InputSameDT=on  OutDataTypeStr=Inherit: Same as first input
  OutPot : Outport
  OutFlow : Outport  Tag=NOFLUX  Port=2
  wires:
  InPot/1 -> OutPot/1  "p_DuplexInverter_test0"
  FlowGain/1 -> OutFlow/1  "f_DuplexInverter_test0"
  FlowSum/1 -> FlowGain/1
  [PushFD2TransmissionHYBPTPlantHybpt_test] -> FlowSum/1
  [PushFD1TransmissionHYBPTPlantHybpt_test] -> FlowSum/2

== system Simple_lib/Driveline/Changan Transmission/LoadScopes/Push ==
  InPot : Inport
  InFlow : Inport  Tag=NOFLUX  Port=2
  OutPot : Outport  Tag=NOFLUX
  tag scope: PushLoadScopesTransmissionHYBPTPlantHybpt_test=global
  wires:
  InFlow/1 -> [PushLoadScopesTransmissionHYBPTPlantHybpt_test]  "flow"
  InPot/1 -> OutPot/1  "pot"

== system Simple_lib/Driveline/Changan Transmission/Shaft1/Pull ==
  InPot : Inport  Tag=NOFLUX
  FlowGain : Gain
  FlowSum : Sum  Inputs=4  SaturateOnIntegerOverflow=on  InputSameDT=on  OutDataTypeStr=Inherit: Same as first input
  OutPot : Outport
  OutFlow : Outport  Tag=NOFLUX  Port=2
  wires:
  InPot/1 -> OutPot/1  "p_DuplexInverter_test0"
  FlowGain/1 -> OutFlow/1  "f_DuplexInverter_test0"
  FlowSum/1 -> FlowGain/1
  [PushGP5TransmissionHYBPTPlantHybpt_test] -> FlowSum/1
  [PushGP1TransmissionHYBPTPlantHybpt_test] -> FlowSum/2
  [PushGP3TransmissionHYBPTPlantHybpt_test] -> FlowSum/3
  [Push_outK1TransmissionHYBPTPlantHybpt_test] -> FlowSum/4

== system Simple_lib/Driveline/Changan Transmission/Shaft2/Pull ==
  InPot : Inport  Tag=NOFLUX
  FlowGain : Gain
  FlowSum : Sum  Inputs=4  SaturateOnIntegerOverflow=on  InputSameDT=on  OutDataTypeStr=Inherit: Same as first input
  OutPot : Outport
  OutFlow : Outport  Tag=NOFLUX  Port=2
  wires:
  InPot/1 -> OutPot/1  "p_DuplexInverter_test0"
  FlowGain/1 -> OutFlow/1  "f_DuplexInverter_test0"
  FlowSum/1 -> FlowGain/1
  [PushGP6TransmissionHYBPTPlantHybpt_test] -> FlowSum/1
  [PushGP2TransmissionHYBPTPlantHybpt_test] -> FlowSum/2
  [PushGP4TransmissionHYBPTPlantHybpt_test] -> FlowSum/3
  [Push_outK2TransmissionHYBPTPlantHybpt_test] -> FlowSum/4

== system Simple_lib/Driveline/Changan Transmission/Synchro/Dynamic Friction ==
  Dw : Inport
  cap : Inport  Port=2
  Product : Product  RndMeth=Zero
  Saturation : Saturate  UpperLimit=inf  LowerLimit=0
  friction : Trigonometry  Operator=tanh
  grab : Gain  Gain=grab
  Tq_dyn : Outport
  wires:
  Dw/1 -> grab/1
  grab/1 -> friction/1
  friction/1 -> Product/2
  cap/1 -> Saturation/1
  Saturation/1 -> Product/1
  Product/1 -> Tq_dyn/1

== system Simple_lib/Driveline/Changan Transmission/Synchro/Push_in ==
  InPot : Inport
  InFlow : Inport  Tag=NOFLUX  Port=2
  OutPot : Outport  Tag=NOFLUX
  tag scope: Push_inSynchroTransmissionHYBPTPlantHybpt_test=global
  wires:
  InPot/1 -> OutPot/1  "pot"
  InFlow/1 -> [Push_inSynchroTransmissionHYBPTPlantHybpt_test]  "flow"

== system Simple_lib/Driveline/Changan Transmission/Synchro/Push_out ==
  InPot : Inport
  InFlow : Inport  Tag=NOFLUX  Port=2
  OutPot : Outport  Tag=NOFLUX
  tag scope: Push_outSynchroTransmissionHYBPTPlantHybpt_test=global
  wires:
  InPot/1 -> OutPot/1  "pot"
  InFlow/1 -> [Push_outSynchroTransmissionHYBPTPlantHybpt_test]  "flow"

== system Simple_lib/Driveline/Changan Transmission/Synchro/Static Friction ==
  cap : Inport
  Dw : Inport  Port=2
  w : Inport  Port=3
  Tq : Inport  Port=4
  1/R2 : Gain  Gain=mu_s/2
  Abs : Abs
  Abs1 : Abs
  Abs2 : Abs
  Delay : Delay  DelayLength=1  InitialCondition=0
  Discrete-Time Integrator : DiscreteIntegrator  gainval=k_static  ExternalReset=level  SampleTime=Ts  ICPrevOutput=DiscIntNeverNeededParam  ICPrevScaledInput=DiscIntNeverNeededParam
  Logical Operator : Logic  Operator=OR  AllPortsSameDT=off  OutDataTypeStr=boolean
  Logical Operator1 : Logic  AllPortsSameDT=off  OutDataTypeStr=boolean
  Logical Operator2 : Logic  Operator=NOT  Inputs=1  AllPortsSameDT=off  OutDataTypeStr=boolean
  Relational Operator : RelationalOperator  OutDataTypeStr=boolean  RndMeth=Nearest
  Relational Operator1 : RelationalOperator  OutDataTypeStr=boolean  RndMeth=Nearest
  Saturation1 : Saturate  UpperLimit=inf  LowerLimit=0
  Sum2 : Sum  Inputs=-++
  big speed diff : Scope
  capacity : Scope
  oldtrans_exceeds_cap : Scope
  slipping : Scope
  Tq_stat : Outport
  wires:
  1/R2/1 -> Relational Operator/2
  Relational Operator/1 -> Logical Operator/1, big speed diff/1
  cap/1 -> capacity/1, Saturation1/1
  Logical Operator/1 -> slipping/1, Discrete-Time Integrator/2
  Discrete-Time Integrator/1 -> Tq_stat/1
  Abs/1 -> Relational Operator/1
  Abs2/1 -> Relational Operator1/1
  Saturation1/1 -> Relational Operator1/2
  Abs1/1 -> 1/R2/1
  Logical Operator1/1 -> oldtrans_exceeds_cap/1, Logical Operator/2
  Sum2/1 -> Abs1/1
  Tq/1 -> Abs2/1
  w/1 -> Sum2/2, Sum2/3
  Dw/1 -> Discrete-Time Integrator/1, Abs/1, Sum2/1
  Relational Operator1/1 -> Delay/1, Logical Operator1/1
  Delay/1 -> Logical Operator2/1
  Logical Operator2/1 -> Logical Operator1/2

== system Simple_lib/Driveline/Changan Transmission/Synchro1/Dynamic Friction ==
  Dw : Inport
  cap : Inport  Port=2
  Product : Product  RndMeth=Zero
  Saturation : Saturate  UpperLimit=inf  LowerLimit=0
  friction : Trigonometry  Operator=tanh
  grab : Gain  Gain=grab
  Tq_dyn : Outport
  wires:
  Dw/1 -> grab/1
  grab/1 -> friction/1
  friction/1 -> Product/2
  cap/1 -> Saturation/1
  Saturation/1 -> Product/1
  Product/1 -> Tq_dyn/1

== system Simple_lib/Driveline/Changan Transmission/Synchro1/Push_in ==
  InPot : Inport
  InFlow : Inport  Tag=NOFLUX  Port=2
  OutPot : Outport  Tag=NOFLUX
  tag scope: Push_inSynchro1TransmissionHYBPTPlantHybpt_test=global
  wires:
  InPot/1 -> OutPot/1  "pot"
  InFlow/1 -> [Push_inSynchro1TransmissionHYBPTPlantHybpt_test]  "flow"

== system Simple_lib/Driveline/Changan Transmission/Synchro1/Push_out ==
  InPot : Inport
  InFlow : Inport  Tag=NOFLUX  Port=2
  OutPot : Outport  Tag=NOFLUX
  tag scope: Push_outSynchro1TransmissionHYBPTPlantHybpt_test=global
  wires:
  InPot/1 -> OutPot/1  "pot"
  InFlow/1 -> [Push_outSynchro1TransmissionHYBPTPlantHybpt_test]  "flow"

== system Simple_lib/Driveline/Changan Transmission/Synchro1/Static Friction ==
  cap : Inport
  Dw : Inport  Port=2
  w : Inport  Port=3
  Tq : Inport  Port=4
  1/R2 : Gain  Gain=mu_s/2
  Abs : Abs
  Abs1 : Abs
  Abs2 : Abs
  Delay : Delay  DelayLength=1  InitialCondition=0
  Discrete-Time Integrator : DiscreteIntegrator  gainval=k_static  ExternalReset=level  SampleTime=Ts  ICPrevOutput=DiscIntNeverNeededParam  ICPrevScaledInput=DiscIntNeverNeededParam
  Logical Operator : Logic  Operator=OR  AllPortsSameDT=off  OutDataTypeStr=boolean
  Logical Operator1 : Logic  AllPortsSameDT=off  OutDataTypeStr=boolean
  Logical Operator2 : Logic  Operator=NOT  Inputs=1  AllPortsSameDT=off  OutDataTypeStr=boolean
  Relational Operator : RelationalOperator  OutDataTypeStr=boolean  RndMeth=Nearest
  Relational Operator1 : RelationalOperator  OutDataTypeStr=boolean  RndMeth=Nearest
  Saturation1 : Saturate  UpperLimit=inf  LowerLimit=0
  Sum2 : Sum  Inputs=-++
  big speed diff : Scope
  capacity : Scope
  oldtrans_exceeds_cap : Scope
  slipping : Scope
  Tq_stat : Outport
  wires:
  1/R2/1 -> Relational Operator/2
  Relational Operator/1 -> Logical Operator/1, big speed diff/1
  cap/1 -> capacity/1, Saturation1/1
  Logical Operator/1 -> slipping/1, Discrete-Time Integrator/2
  Discrete-Time Integrator/1 -> Tq_stat/1
  Abs/1 -> Relational Operator/1
  Abs2/1 -> Relational Operator1/1
  Saturation1/1 -> Relational Operator1/2
  Abs1/1 -> 1/R2/1
  Logical Operator1/1 -> oldtrans_exceeds_cap/1, Logical Operator/2
  Sum2/1 -> Abs1/1
  Tq/1 -> Abs2/1
  w/1 -> Sum2/2, Sum2/3
  Dw/1 -> Discrete-Time Integrator/1, Abs/1, Sum2/1
  Relational Operator1/1 -> Delay/1, Logical Operator1/1
  Delay/1 -> Logical Operator2/1
  Logical Operator2/1 -> Logical Operator1/2

== system Simple_lib/Driveline/Changan Transmission/Synchro2/Dynamic Friction ==
  Dw : Inport
  cap : Inport  Port=2
  Product : Product  RndMeth=Zero
  Saturation : Saturate  UpperLimit=inf  LowerLimit=0
  friction : Trigonometry  Operator=tanh
  grab : Gain  Gain=grab
  Tq_dyn : Outport
  wires:
  Dw/1 -> grab/1
  grab/1 -> friction/1
  friction/1 -> Product/2
  cap/1 -> Saturation/1
  Saturation/1 -> Product/1
  Product/1 -> Tq_dyn/1

== system Simple_lib/Driveline/Changan Transmission/Synchro2/Push_in ==
  InPot : Inport
  InFlow : Inport  Tag=NOFLUX  Port=2
  OutPot : Outport  Tag=NOFLUX
  tag scope: Push_inSynchro2TransmissionHYBPTPlantHybpt_test=global
  wires:
  InPot/1 -> OutPot/1  "pot"
  InFlow/1 -> [Push_inSynchro2TransmissionHYBPTPlantHybpt_test]  "flow"
